simulink library "martin_sean_RoombaLib"  (R2017a)
settings: Solver=VariableStepAuto  StartTime=0.0  StopTime=10.0  RelTol=1e-3
settings Model: Creator=tuf53749  LastModifiedBy=Sean

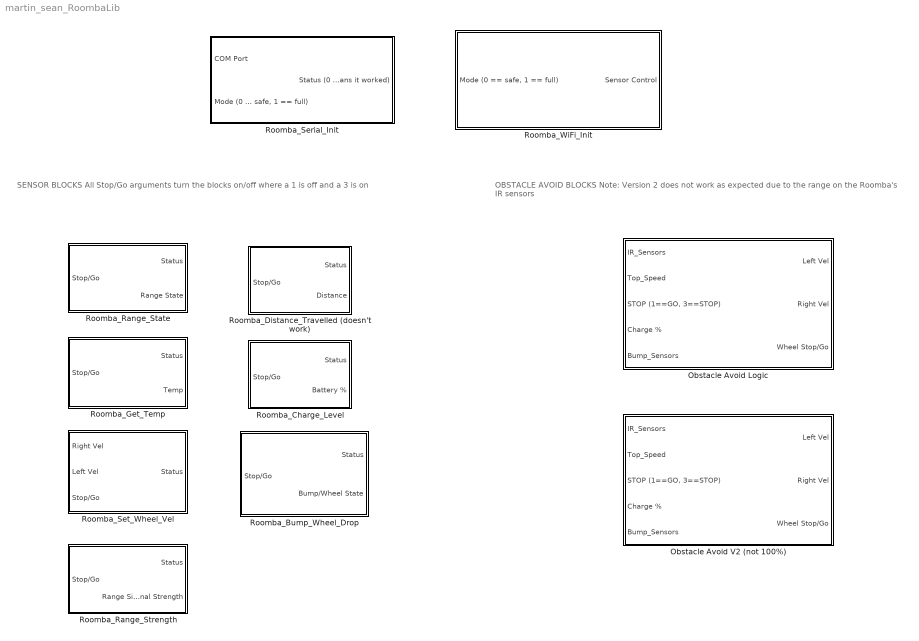
== system martin_sean_RoombaLib ==
  note: OBSTACLE AVOID BLOCKS
      |
      | Note: Version 2 does not work as expected due to the range on the Roomba's IR sensors
  note: SENSOR BLOCKS
      |
      | All Stop/Go arguments turn the blocks on/off where a 1 is off and a 3 is on
  Obstacle Avoid Logic : Subsystem
  Obstacle Avoid V2 (not 100%) : Subsystem
  Roomba_Bump_Wheel_Drop : Subsystem
  Roomba_Charge_Level : Subsystem  Description=Returns the battery charge level on the Roomba as a percentage. Updates every 100 seconds.  mask(Charge Level Roomba){}
      mask help: Returns the battery charge level on the Roomba as a percentage. Updates every 100 seconds.
  Roomba_Distance_Travelled (doesn't work) : Subsystem  mask(Distance Travelled Roomba){}
      mask help: Takes in the counts from the Roomba's wheel encoders. Using the diameter of the wheels this value is manipulated to obtain a distance the wheels have spun. STILL NEEDS TO BE FINISHED.
  Roomba_Get_Temp : Subsystem  Description=|  mask(Get Temperature Roomba){}
      | Returns the value of the temperature sensor on the Roomba in degrees Celcius. Updates every
      | 30 seconds.
      mask help: Returns the value of the temperature sensor on the Roomba in degrees Celcius. Updates every 30 seconds.
  Roomba_Range_State : Subsystem  Description=|  mask(Range State Roomba){}
      | Returns [1x6] array containing the state of the six IR sensors on the front of the Roomba. A 
      | '1' indicates there is an object ahead and a '0' indicates no object.
      mask help:
      | Returns [1x6] array containing the state of the six IR sensors on the front of the Roomba. A
      | '1' indicates there is an object ahead and a '0' indicates no object.
  Roomba_Range_Strength : Subsystem  Description=|  mask(Range State Roomba){}
      | Returns [1x6] array containing the state of the six IR sensors on the front of the Roomba. A 
      | '1' indicates there is an object ahead and a '0' indicates no object.
      mask help:
      | Returns [1x6] array containing the state of the six IR sensors on the front of the Roomba. A
      | '1' indicates there is an object ahead and a '0' indicates no object.
  Roomba_Serial_Init : Subsystem  Description=|  Priority=-1000  StartFcn=|  StopFcn=|  mask(Roomba Serial Port Initialization){}
      Description=|
      | Initializes a serial connection to the Roomba. Takes the COM Port number and mode as inputs.
      | For instance, COM Port = 3 and Mode = 1 will set up a connection to the Roomba on COM3
      | and place it in 'full' mode.
      | 
      | A 0 is returned after successful initialization.
      StartFcn=|
      | %clear the workspace of old Roomba obj
      | clear all;
      StopFcn=|
      | %this sends a reset and stop cmd to the 
      | %Roomba before quiting sim
      | coder.extrinsic('RoombaClose');
      | RoombaClose;
      mask help:
      | Initializes a serial connection to the Roomba. Takes the COM Port number and mode as inputs.
      | For instance, COM Port = 3 and Mode = 1 will set up a connection to the Roomba on COM3
      | and place it in 'full' mode.
      |
      | A 0 is returned after successful initialization.
  Roomba_Set_Wheel_Vel : Subsystem  Description=|  mask(Set Wheel Velocity Roomba){}
      | Sets the right and left wheel velocities on the Roomba. The values are in meters/sec between 
      | [-0.5, 0.5]. Negative velocity is backwards.
      mask help: Sets the right and left wheel velocities on the Roomba. The values are in meters/sec between [-0.5, 0.5]. Negative velocity is backwards.
  Roomba_WiFi_Init : Subsystem  Description=|  Priority=-1000  StartFcn=|  StopFcn=|  mask(Roomba WiFi Initialization){}
      Description=|
      | Initializes a WiFi connection to the Roomba. The RooWiFi module is used. Takes the mode as an
      | input. For instance, Mode = 1 will set up a connection to the Roomba over RooWiFi on 10.0.0.1
      | and place it in 'full' mode.
      | 
      | A 0 is returned after successful initialization.
      | 
      | RooWiFi documentation:
      | http://www.roowifi.com/wp-content/uploads/RwRemote_User_Guide_v2_rev15.pdf
      StartFcn=|
      | %clear the workspace of old Roomba obj
      | clear all;
      StopFcn=|
      | %this sends a reset and stop cmd to the 
      | %Roomba before quiting sim
      | coder.extrinsic('RoombaClose');
      | RoombaClose;
      | clear all;
      mask help:
      | Initializes a WiFi connection to the Roomba. The RooWiFi module is used. Takes the mode as an
      | input. For instance, Mode = 1 will set up a connection to the Roomba over RooWiFi on 10.0.0.1
      | and place it in 'full' mode.
      |
      | A 0 is returned after successful initialization.
      |
      | RooWiFi documentation:
      | http://www.roowifi.com/wp-content/uploads/RwRemote_User_Guide_v2_rev15.pdf

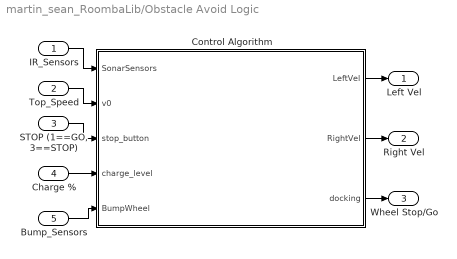
== system martin_sean_RoombaLib/Obstacle Avoid Logic ==
  IR_Sensors : Inport
  Top_Speed : Inport  Port=2
  "STOP (1==GO, 3==STOP)" : Inport  Port=3
  Charge % : Inport  Port=4
  Bump_Sensors : Inport  Port=5
  Control Algorithm : Stateflow chart  TreatAsAtomicUnit=on  mask{v0=1}
      mask prompts: v0 "Wheel Angular Velocity"
  Left Vel : Outport
  Right Vel : Outport  Port=2
  Wheel Stop/Go : Outport  Port=3
  wires:
  "STOP (1==GO, 3==STOP)"/1 -> Control Algorithm/3(stop_button)
  Charge %/1 -> Control Algorithm/4(charge_level)
  Bump_Sensors/1 -> Control Algorithm/5(BumpWheel)
  Control Algorithm/3(docking) -> Wheel Stop/Go/1
  Control Algorithm/2(RightVel) -> Right Vel/1
  Control Algorithm/1(LeftVel) -> Left Vel/1
  IR_Sensors/1 -> Control Algorithm/1(SonarSensors)
  Top_Speed/1 -> Control Algorithm/2(v0)

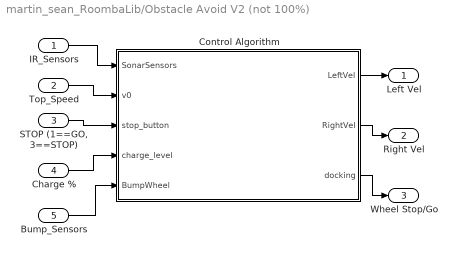
== system martin_sean_RoombaLib/Obstacle Avoid V2 (not 100%) ==
  IR_Sensors : Inport
  Top_Speed : Inport  Port=2
  "STOP (1==GO, 3==STOP)" : Inport  Port=3
  Charge % : Inport  Port=4
  Bump_Sensors : Inport  Port=5
  Control Algorithm : Stateflow chart  TreatAsAtomicUnit=on  mask{v0=1}
      mask prompts: v0 "Wheel Angular Velocity"
  Left Vel : Outport
  Right Vel : Outport  Port=2
  Wheel Stop/Go : Outport  Port=3
  wires:
  "STOP (1==GO, 3==STOP)"/1 -> Control Algorithm/3(stop_button)
  Charge %/1 -> Control Algorithm/4(charge_level)
  Bump_Sensors/1 -> Control Algorithm/5(BumpWheel)
  Control Algorithm/3(docking) -> Wheel Stop/Go/1
  Control Algorithm/2(RightVel) -> Right Vel/1
  Control Algorithm/1(LeftVel) -> Left Vel/1
  IR_Sensors/1 -> Control Algorithm/1(SonarSensors)
  Top_Speed/1 -> Control Algorithm/2(v0)

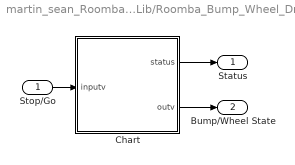
== system martin_sean_RoombaLib/Roomba_Bump_Wheel_Drop ==
  Stop/Go : Inport
  Chart : Stateflow chart  TreatAsAtomicUnit=on
  Status : Outport
  Bump/Wheel State : Outport  Port=2
  wires:
  Stop/Go/1 -> Chart/1(inputv)
  Chart/1(status) -> Status/1
  Chart/2(outv) -> Bump/Wheel State/1

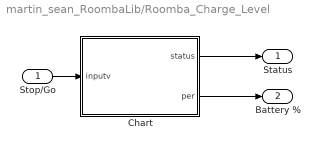
== system martin_sean_RoombaLib/Roomba_Charge_Level ==
  Stop/Go : Inport
  Chart : Stateflow chart  TreatAsAtomicUnit=on
  Status : Outport
  Battery % : Outport  Port=2
  wires:
  Stop/Go/1 -> Chart/1(inputv)
  Chart/1(status) -> Status/1
  Chart/2(per) -> Battery %/1

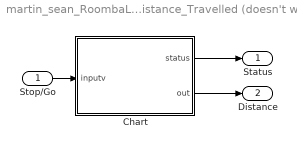
== system martin_sean_RoombaLib/Roomba_Distance_Travelled (doesn't work) ==
  Stop/Go : Inport
  Chart : Stateflow chart  TreatAsAtomicUnit=on
  Status : Outport
  Distance : Outport  Port=2
  wires:
  Chart/2(out) -> Distance/1
  Stop/Go/1 -> Chart/1(inputv)
  Chart/1(status) -> Status/1

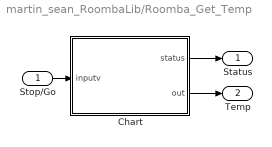
== system martin_sean_RoombaLib/Roomba_Get_Temp ==
  Stop/Go : Inport
  Chart : Stateflow chart  TreatAsAtomicUnit=on
  Status : Outport
  Temp : Outport  Port=2
  wires:
  Stop/Go/1 -> Chart/1(inputv)
  Chart/1(status) -> Status/1
  Chart/2(out) -> Temp/1

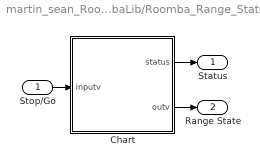
== system martin_sean_RoombaLib/Roomba_Range_State ==
  Stop/Go : Inport
  Chart : Stateflow chart  TreatAsAtomicUnit=on
  Status : Outport
  Range State : Outport  Port=2
  wires:
  Chart/1(status) -> Status/1
  Chart/2(outv) -> Range State/1
  Stop/Go/1 -> Chart/1(inputv)

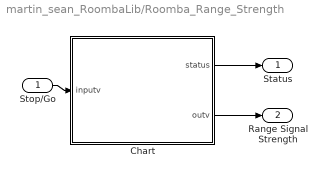
== system martin_sean_RoombaLib/Roomba_Range_Strength ==
  Stop/Go : Inport
  Chart : Stateflow chart  TreatAsAtomicUnit=on
  Status : Outport
  Range Signal Strength : Outport  Port=2
  wires:
  Chart/1(status) -> Status/1
  Chart/2(outv) -> Range Signal Strength/1
  Stop/Go/1 -> Chart/1(inputv)

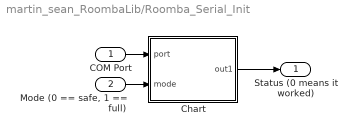
== system martin_sean_RoombaLib/Roomba_Serial_Init ==
  COM Port : Inport
  "Mode (0 == safe, 1 == full)" : Inport  Port=2
  Chart : Stateflow chart  TreatAsAtomicUnit=on
  Status (0 means it worked) : Outport
  wires:
  COM Port/1 -> Chart/1(port)
  "Mode (0 == safe, 1 == full)"/1 -> Chart/2(mode)
  Chart/1(out1) -> Status (0 means it worked)/1

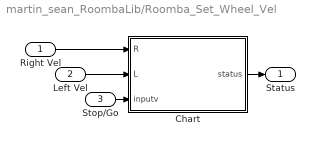
== system martin_sean_RoombaLib/Roomba_Set_Wheel_Vel ==
  Right Vel : Inport  OutMin=[-0.5]  OutMax=[0.5]
  Left Vel : Inport  Port=2  OutMin=[-0.5]  OutMax=[0.5]
  Stop/Go : Inport  Port=3
  Chart : Stateflow chart  TreatAsAtomicUnit=on
  Status : Outport
  wires:
  Right Vel/1 -> Chart/1(R)
  Left Vel/1 -> Chart/2(L)
  Chart/1(status) -> Status/1
  Stop/Go/1 -> Chart/3(inputv)

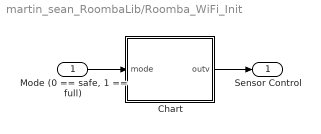
== system martin_sean_RoombaLib/Roomba_WiFi_Init ==
  "Mode (0 == safe, 1 == full)" : Inport
  Chart : Stateflow chart  TreatAsAtomicUnit=on
  "Sensor Control " : Outport
  wires:
  "Mode (0 == safe, 1 == full)"/1 -> Chart/1(mode)
  Chart/1(outv) -> "Sensor Control "/1

== system martin_sean_RoombaLib/Obstacle Avoid Logic/Control Algorithm/EmergencyStopLogic.stop ==
  f : TriggerPort  TriggerType=function-call  VariantControl=(inherit)
      settings: CopyFcn=Stateflow.SLINSF.SimulinkMan.removeBlockPreDeleteFcn  PreDeleteFcn=Stateflow.SLINSF.SimulinkMan.unsafePredeleteFcn
  Constant : Constant
  Stop Simulation : Stop
  wires:
  Constant/1 -> Stop Simulation/1

== system martin_sean_RoombaLib/Obstacle Avoid V2 (not 100%)/Control Algorithm/EmergencyStopLogic.stop ==
  f : TriggerPort  TriggerType=function-call  VariantControl=(inherit)
      settings: CopyFcn=Stateflow.SLINSF.SimulinkMan.removeBlockPreDeleteFcn  PreDeleteFcn=Stateflow.SLINSF.SimulinkMan.unsafePredeleteFcn
  Constant : Constant
  Stop Simulation : Stop
  wires:
  Constant/1 -> Stop Simulation/1

== stateflow chart martin_sean_RoombaLib/Roomba_Range_State/Chart ==
  state Init_Vector
    en:
    outv = [0,0,0,0,0,0];
    status=0;
  state Limbo
    en,du:
    outv=RangeStateRoomba_Get;
    status=2;
  state NoCommand
    en:
    outv = [0,0,0,0,0,0];
    status=1;
  (default) -> Init_Vector
  Init_Vector -> NoCommand
  NoCommand -> Limbo : [inputv==3]
  Limbo -> NoCommand : [inputv==1]
  data: y function_output; status output; outv output; inputv input
  function y = RangeStateRoomba_Get:
    | function y = RangeStateRoomba_Get
    | persistent obj
    | y = [0,0,0,0,0,0];
    | coder.extrinsic('RangeStateRoomba');
    | coder.extrinsic('evalin');
    | coder.extrinsic('get');
    | if isempty(obj)
    |     obj = evalin('base','objWs');
    | end
    | y = RangeStateRoomba(obj);

== stateflow chart martin_sean_RoombaLib/Roomba_Set_Wheel_Vel/Chart ==
  state StoppedWheels
    en:
    SetWheelVelRoomba_Get(0,0);
    status=0;
  state Limbo
    en:
    SetWheelVelRoomba_Get(R,L);
    status=1;
  (default) -> StoppedWheels
  Limbo -> StoppedWheels [order 1] : [inputv==1]
  StoppedWheels -> Limbo : [inputv==3]
  Limbo -> Limbo [order 2] : after(0.0001,sec)
  data: right function_input [-0.5..0.5]; left function_input [-0.5..0.5]; status output; R input [-0.5..0.5]; L input [-0.5..0.5]; inputv input
  function SetWheelVelRoomba_Get(right,left):
    | function SetWheelVelRoomba_Get(right,left)
    | persistent obj
    | coder.extrinsic('SetWheelVelRoomba');
    | coder.extrinsic('evalin');
    | coder.extrinsic('get');
    | if isempty(obj)
    |     obj = evalin('base','objWs');
    | end
    | y = SetWheelVelRoomba(obj,right,left);

== stateflow chart martin_sean_RoombaLib/Roomba_Serial_Init/Chart ==
  state State
    en,du:
    serial_Init(port,mode);
    out1 = 0;
  (default) -> State
  data: x function_input; y function_input; port input; out1 output; mode input
  function serial_Init(x,y):
    | function serial_Init(x,y)
    | coder.extrinsic('RoombaInit');
    | coder.extrinsic('num2str');
    | coder.extrinsic('strcat');
    | coder.extrinsic('instrreset');
    | coder.extrinsic('instrfind');
    | coder.extrinsic('delete');
    | coder.extrinsic('serial');
    | coder.extrinsic('assignin');
    | persistent obj
    | mode_string = 'safe';
    | if isempty(obj)
    |     if y == 1
    |         mode_string = 'full';
    |     end
    |     obj=RoombaInit(x,mode_string);
    |     assignin('base','objWs',obj);
    | end

== stateflow chart martin_sean_RoombaLib/Roomba_WiFi_Init/Chart ==
  state State
    en,du:
    outv=1;
    Sensor_Control = wifi_Init(mode);
  state StartSensor
    en,du:
    outv=3;
  (default) -> State : {Sensor_Control = 0;}
  State -> StartSensor : [Sensor_Control==1 && after(5,sec)]
  data: y function_input; x function_output; mode input; Sensor_Control local; outv output
  function x = wifi_Init(y):
    | function x = wifi_Init(y)
    | x = 1;
    | coder.extrinsic('RoombaInit_tcp');
    | coder.extrinsic('num2str');
    | coder.extrinsic('strcat');
    | coder.extrinsic('instrreset');
    | coder.extrinsic('instrfind');
    | coder.extrinsic('delete');
    | coder.extrinsic('serial');
    | coder.extrinsic('assignin');
    | persistent obj
    | mode_string = 'safe';
    | if isempty(obj)
    |     if y == 1
    |         mode_string = 'full';
    |     end
    |     obj=RoombaInit_tcp('10.0.0.1',mode_string);
    |     assignin('base','objWs',obj);
    | end

== stateflow chart martin_sean_RoombaLib/Roomba_Get_Temp/Chart ==
  state StoppedWheels
    en:
    out = nan;
    status=0;
  state Limbo
    en:
    out = RoombaTemperature_Get;
    status=1;
  (default) -> StoppedWheels
  Limbo -> StoppedWheels [order 1] : [inputv==1]
  StoppedWheels -> Limbo : [inputv==3]
  Limbo -> Limbo [order 2] : after(30,sec)
  data: y function_output; status output; inputv input; out output
  function y = RoombaTemperature_Get:
    | function y = RoombaTemperature_Get
    | persistent obj
    | coder.extrinsic('TemperatureRoomba');
    | coder.extrinsic('evalin');
    | coder.extrinsic('get');
    | if isempty(obj)
    |     obj = evalin('base','objWs');
    | end
    | y = TemperatureRoomba(obj);

== stateflow chart martin_sean_RoombaLib/Roomba_Distance_Travelled (doesn't work)/Chart ==
  state ResetStart
    en:
    out = 0;
    status=0;
  state Limbo
    en:
    counts = EncoderSensorsRoomba_Get;
    out = counts*pi*2*0.036/508.8;
    status=1;
  (default) -> ResetStart
  Limbo -> ResetStart [order 1] : [inputv==1]
  ResetStart -> Limbo : [inputv==3]
  Limbo -> Limbo [order 2] : after(0.1,sec)
  data: y function_output; status output; inputv input; out output; counts local
  function y = EncoderSensorsRoomba_Get:
    | function y = EncoderSensorsRoomba_Get
    | persistent obj
    | coder.extrinsic('TemperatureRoomba');
    | coder.extrinsic('evalin');
    | coder.extrinsic('get');
    | if isempty(obj)
    |     obj = evalin('base','objWs');
    | end
    | y = TemperatureRoomba(obj);

== stateflow chart martin_sean_RoombaLib/Roomba_Charge_Level/Chart ==
  state ResetStart
    en:
    per = nan;
    status=0;
  state Limbo
    en:
    [charge,cap,per] = BatteryChargeReaderRoomba_Get;
    status=1;
  (default) -> ResetStart
  ResetStart -> Limbo : [inputv==3]
  Limbo -> ResetStart [order 1] : [inputv==1]
  Limbo -> Limbo [order 2] : after(100,sec)
  data: x function_output; y function_output; z function_output; status output; inputv input; charge local; per output; cap local
  function [x,y,z] = BatteryChargeReaderRoomba_Get:
    | function [x,y,z] = BatteryChargeReaderRoomba_Get
    | persistent obj
    | coder.extrinsic('BatteryChargeReaderRoomba');
    | coder.extrinsic('evalin');
    | coder.extrinsic('get');
    | if isempty(obj)
    |     obj = evalin('base','objWs');
    | end
    | [x,y,z] = BatteryChargeReaderRoomba(obj);

== stateflow chart martin_sean_RoombaLib/Obstacle Avoid Logic/Control Algorithm ==
  state EmergencyStopLogic [parallel]
    settings: executionOrder=3
    state StopButtonOFF
      en:
      %do nothing
      %
    state stop [function]
    state StopButtonON
      en:
      docking = 3;
      LeftVel = 0;
      RightVel = 0;
      %call stop sim block
      %
      stop;
    (default) -> StopButtonOFF
    StopButtonOFF -> StopButtonON : [stop_button == 3]
  state ObstacleAvoidLogic [parallel]
    en,du:
    left=[SonarSensors(1:3)]
    right=[SonarSensors(4:6)]
    sensors = [left,right];
    rightbump=[BumpWheel(1)];
    leftbump=[BumpWheel(2)];
    bothbump=[BumpWheel(3)];
    %LWheelDrop=[BumpWheel(4)];
    %RWheelDrop=[BumpWheel(5)];
    settings: executionOrder=1
    state InitialCount
      en:
      count=0;
    state ReverseABit
      en,du:
      RightVel = -v0;
      LeftVel = -v0;
    state GoStraight
      en,du:
      RightVel = v0;
      LeftVel = v0;
    state STOP
      du :
      RightVel = 0;
      LeftVel = 0;
    state DetermineRightLeft
    state ReverseRight
      en,du:
      RightVel = -v0;
      LeftVel = -v0;
    state ReverseLeft
      en,du:
      RightVel = -v0;
      LeftVel = -v0;
    state TurnLeftInPlace1
      du :
      RightVel = v0;
      LeftVel = -v0;
    state Reverse
      en,du:
      RightVel = -v0;
      LeftVel = -v0;
    state TurnRightInPlace1
      du :
      RightVel = -v0;
      LeftVel = v0;
    state TurnLeftInPlace
      du :
      RightVel = v0;
      LeftVel = -v0;
    state TurnRightInPlace
      du :
      RightVel = -v0;
      LeftVel = v0;
    (default) -> InitialCount
    InitialCount -> ReverseABit
    ReverseABit -> GoStraight : after(1,sec)
    TurnLeftInPlace -> GoStraight : [all(right<1) && after(0.5,sec)]
    GoStraight -> STOP [order 1] : [any(sensors == 1)]
    TurnRightInPlace -> GoStraight : [all(left<1) && after(0.5,sec)]
    GoStraight -> Reverse [order 2] : [bothbump==1]
    Reverse -> GoStraight : after(0.5,sec)
    GoStraight -> ReverseRight [order 3] : [leftbump==1]
    TurnRightInPlace1 -> GoStraight : [all(left<1) && after(0.5,sec)]
    GoStraight -> ReverseLeft [order 4] : [rightbump==1]
    TurnLeftInPlace1 -> GoStraight : [all(right<1) && after(0.5,sec)]
    STOP -> DetermineRightLeft : after(0.5,sec)
    ReverseLeft -> TurnLeftInPlace1 : after(0.5,sec)
    ReverseRight -> TurnRightInPlace1 : after(0.5,sec)
    DetermineRightLeft -> TurnLeftInPlace [order 2] : %default
    DetermineRightLeft -> TurnRightInPlace [order 1] : [any(left) == 1]
  state BatteryLevelLogic [parallel]
    settings: executionOrder=2
    state START
    state CheckBat
      en:
      docking = 3;
    state LowBat
      en:
      docking = 1;
      SeekDockRoomba_Get();
    (default) -> START
    START -> CheckBat : after(5,sec)
    CheckBat -> LowBat : [charge_level <= 10]
  data: LeftVel output; RightVel output; SonarSensors input; v0 input [0..0.5]; stop_button input; charge_level input; docking output; front local; BumpWheel input; LWheelDrop local; RWheelDrop local; rightbump local; leftbump local; bothbump local; right local; sensors local; left local; count local
  function SeekDockRoomba_Get:
    | function SeekDockRoomba_Get
    | persistent obj
    | coder.extrinsic('SeekDockRoomba');
    | coder.extrinsic('evalin');
    | coder.extrinsic('get');
    | if isempty(obj)
    |     obj = evalin('base','objWs');
    | end
    | SeekDockRoomba(obj);

== stateflow chart martin_sean_RoombaLib/Roomba_Bump_Wheel_Drop/Chart ==
  state Init_Vector
    en:
    outv = [nan,nan,nan,nan,nan];
    status=0;
  state Limbo
    en,du:
    [outv(1),outv(2),outv(3),outv(4),outv(5)]=BumperRoomba_Get;
    status=2;
  state NoCommand
    en:
    outv = [nan,nan,nan,nan,nan];
    status=1;
  (default) -> Init_Vector
  Init_Vector -> NoCommand
  NoCommand -> Limbo : [inputv==3]
  Limbo -> NoCommand : [inputv==1]
  data: a function_output; b function_output; c function_output; d function_output; e function_output; status output; outv output; inputv input
  function [a,b,c,d,e] = BumperRoomba_Get:
    | function [a,b,c,d,e] = BumperRoomba_Get
    | persistent obj
    | a=nan;b=nan;c=nan;d=nan;e=nan;
    | coder.extrinsic('BumpsWheelDropsSensorsRoomba');
    | coder.extrinsic('evalin');
    | coder.extrinsic('get');
    | if isempty(obj)
    |     obj = evalin('base','objWs');
    | end
    | [a,b,c,d,e] = BumpsWheelDropsSensorsRoomba(obj);

== stateflow chart martin_sean_RoombaLib/Roomba_Range_Strength/Chart ==
  state Init_Vector
    en:
    outv = [nan,nan,nan,nan,nan,nan];
    status=0;
  state Limbo
    en,du:
    outv=RangeSignalStrengthRoomba_Get();
    status=2;
  state NoCommand
    en:
    outv = [nan,nan,nan,nan,nan,nan];
    status=1;
  (default) -> Init_Vector
  Init_Vector -> NoCommand
  NoCommand -> Limbo : [inputv==3]
  Limbo -> NoCommand : [inputv==1]
  data: y function_output; status output; outv output; inputv input
  function y = RangeSignalStrengthRoomba_Get:
    | function y = RangeSignalStrengthRoomba_Get
    | persistent obj
    | y = [0,0,0,0,0,0];
    | coder.extrinsic('RangeSignalStrengthRoomba');
    | coder.extrinsic('evalin');
    | coder.extrinsic('get');
    | if isempty(obj)
    |     obj = evalin('base','objWs');
    | end
    | y = RangeSignalStrengthRoomba(obj);

== stateflow chart martin_sean_RoombaLib/Obstacle Avoid V2 (not 100%)/Control Algorithm ==
  state EmergencyStopLogic [parallel]
    settings: executionOrder=3
    state StopButtonOFF
      en:
      %do nothing
      %
    state stop [function]
    state StopButtonON
      en:
      docking = 3;
      LeftVel = 0;
      RightVel = 0;
      %call stop sim block
      %
      stop;
    (default) -> StopButtonOFF
    StopButtonOFF -> StopButtonON : [stop_button == 3]
  state ObstacleAvoidLogic [parallel]
    en,du:
    leftMT=[SonarSensors(1)];
    leftMD=[SonarSensors(2)];
    leftFT=[SonarSensors(3)];
    rightFT=[SonarSensors(4)];
    rightMD=[SonarSensors(5)];
    rightMT=[SonarSensors(6)];
    front = [leftFT,rightFT];
    rightbump=[BumpWheel(1)];
    leftbump=[BumpWheel(2)];
    bothbump=[BumpWheel(3)];
    %LWheelDrop=[BumpWheel(4)];
    %RWheelDrop=[BumpWheel(5)];
    settings: executionOrder=1
    state InitialCount
      en:
      count=0;
    state ReverseABit
      en,du:
      RightVel = -v0;
      LeftVel = -v0;
    state GoStraight
      en,du:
      RightVel = v0;
      LeftVel = v0;
    state DetermineRightLeft
    state Reverse
      en,du:
      RightVel = -v0;
      LeftVel = -v0;
    state ReverseRight
      en,du:
      RightVel = -v0;
      LeftVel = -v0;
    state ReverseLeft
      en,du:
      RightVel = -v0;
      LeftVel = -v0;
    state TurnRightWide
      du:
      RightVel = v0/2;
      LeftVel = v0;
    state TurnRightTight
      du :
      RightVel = v0/5;
      LeftVel = v0;
    state TurnLeftInPlace
      du :
      RightVel = v0;
      LeftVel = -v0;
    state TurnRightInPlace
      du :
      RightVel = -v0;
      LeftVel = v0;
    state TurnLeftTight
      du :
      RightVel = v0;
      LeftVel = v0/5;
    state TurnLeftWide
      du :
      RightVel = v0;
      LeftVel = v0/2;
    state TurnRightInPlace1
      du :
      RightVel = -v0;
      LeftVel = v0;
    state TurnLeftInPlace1
      du :
      RightVel = v0;
      LeftVel = -v0;
    (default) -> InitialCount
    InitialCount -> ReverseABit
    ReverseABit -> GoStraight : after(3,sec)
    TurnRightInPlace1 -> GoStraight : [all(front<1) && after(0.5,sec)]
    TurnLeftInPlace1 -> GoStraight : [all(front<1) && after(0.5,sec)]
    GoStraight -> TurnRightWide [order 3] : [leftMT==1&&all(front<1)]
    TurnRightWide -> GoStraight : [leftMT<1]
    GoStraight -> TurnRightTight [order 2] : [leftMD==1&&...
        | all(front<1)]
    TurnRightTight -> GoStraight : [leftMT<1&&leftMD<1]
    TurnLeftInPlace -> GoStraight : [all(front<1) && after(0.5,sec)]
    TurnRightInPlace -> GoStraight : [all(front<1) && after(0.5,sec)]
    GoStraight -> TurnLeftTight [order 4] : [rightMD==1&&...
        | all(front<1)]
    TurnLeftTight -> GoStraight : [rightMD<1&&rightMT<1]
    GoStraight -> TurnLeftWide [order 5] : [rightMT==1&&all(front<1)]
    TurnLeftWide -> GoStraight : [rightMT<1]
    Reverse -> GoStraight : after(3,sec)
    GoStraight -> DetermineRightLeft [order 1] : [any(front == 1)]
    GoStraight -> Reverse [order 6] : [bothbump==1]
    GoStraight -> ReverseRight [order 7] : [leftbump==1]
    GoStraight -> ReverseLeft [order 8] : [rightbump==1]
    DetermineRightLeft -> TurnLeftInPlace [order 2] : %default
    DetermineRightLeft -> TurnRightInPlace [order 1] : [leftFT == 1]
    ReverseRight -> TurnRightInPlace1 : after(3,sec)
    ReverseLeft -> TurnLeftInPlace1 : after(3,sec)
  state BatteryLevelLogic [parallel]
    settings: executionOrder=2
    state CheckBat
      en:
      docking = 3;
    state LowBat
      en:
      docking = 1;
      SeekDockRoomba_Get();
    (default) -> CheckBat
    CheckBat -> LowBat : [charge_level <= 10]
  data: LeftVel output; RightVel output; SonarSensors input; frontSensors local; leftMostSensors local; leftMiddleSensors local; rightMostSensors local; rightMiddleSensors local; rightMT local; leftFT local; rightMD local; rightFT local; leftMD local; leftMT local; count local; v0 input [0..0.5]; stop_button input; charge_level input; docking output; front local; BumpWheel input; LWheelDrop local; RWheelDrop local; rightbump local; leftbump local; bothbump local
  function SeekDockRoomba_Get:
    | function SeekDockRoomba_Get
    | persistent obj
    | coder.extrinsic('SeekDockRoomba');
    | coder.extrinsic('evalin');
    | coder.extrinsic('get');
    | if isempty(obj)
    |     obj = evalin('base','objWs');
    | end
    | SeekDockRoomba(obj);
